simulink library "Qnorm"  (R2014b)
settings: Solver=ode45  StartTime=0.0  StopTime=10.0  RelTol=1e-3
settings Model: Creator=Hp  LastModifiedBy=Hp

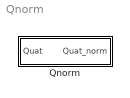
== system Qnorm ==
  Qnorm : Subsystem

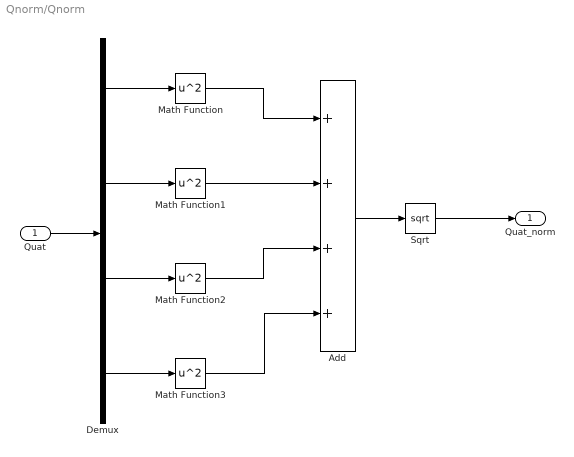
== system Qnorm/Qnorm ==
  Quat : Inport
  Add : Sum  Inputs=++++
  Demux : Demux
  Math Function{,1..3} (4 alike) : Math  Operator=square  SaturateOnIntegerOverflow=on
  Sqrt : Sqrt  SaturateOnIntegerOverflow=on
  Quat_norm : Outport
  wires:
  Quat/1 -> Demux/1
  Demux/2 -> Math Function1/1
  Sqrt/1 -> Quat_norm/1
  Demux/4 -> Math Function3/1
  Demux/1 -> Math Function/1
  Demux/3 -> Math Function2/1
  Math Function1/1 -> Add/2
  Math Function3/1 -> Add/4
  Add/1 -> Sqrt/1
  Math Function/1 -> Add/1
  Math Function2/1 -> Add/3
